simulink model "uav_with_flc_optimized_by_ga"  (R2025b)
settings: Solver=ode45  StartTime=0.0  StopTime=30  FixedStep=0.01  RelTol=1e-3
undefined symbols (not defined in the file): Ax, Ay, Az, b, d, g, Ixx, Iyy, Izz, Jr, k1_phi, k1_psi, k1_theta, k1_x, k1_y, k1_z, k2_phi, k2_psi, k2_theta, k2_x, k2_y, k2_z, Kout_phi, Kout_theta, Kout_x, Kout_y, Kout_z, L, m, omega_max, phi_ref_max, theta_ref_max, U1_max, U1_min, U2_max, U3_max, U4_max
libraries: fuzblock x6
settings Model: SimulationMode=accelerator  Creator=pc  LastModifiedBy=pc

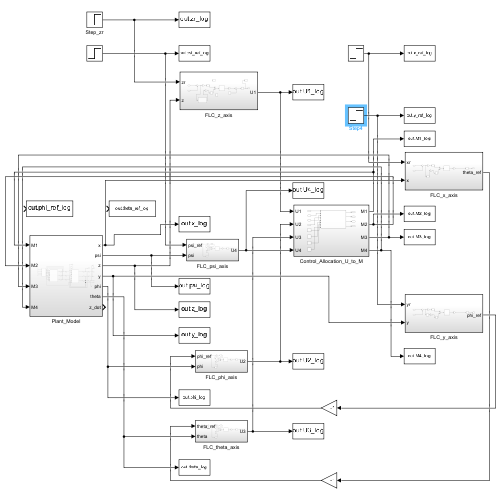
[thumbnail: Simulink's stored preview of the top-level diagram]
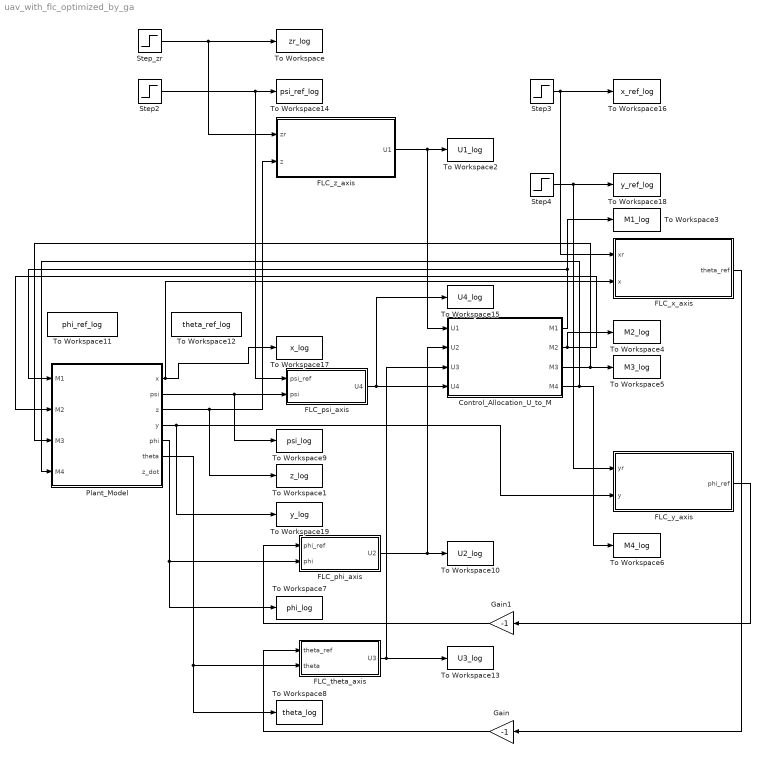
== system uav_with_flc_optimized_by_ga ==
  Control_Allocation_U_to_M : Subsystem
  FLC_phi_axis : Subsystem
  FLC_psi_axis : Subsystem
  FLC_theta_axis : Subsystem
  FLC_x_axis : Subsystem
  FLC_y_axis : Subsystem
  FLC_z_axis : Subsystem
  Gain : Gain  Gain=-1
  Gain1 : Gain  Gain=-1
  Plant_Model : Subsystem
  Step2 : Step  Time=5  After=0  SampleTime=0
  Step3 : Step  Time=10  After=0.2  SampleTime=0
  Step4 : Step  Time=10  After=0.2  SampleTime=0
  Step_zr : Step  SampleTime=0
  To Workspace : ToWorkspace  VariableName=zr_log  SaveFormat=Timeseries  SampleTime=-1
  To Workspace1 : ToWorkspace  VariableName=z_log  SaveFormat=Timeseries  SampleTime=-1
  To Workspace10 : ToWorkspace  VariableName=U2_log  SaveFormat=Timeseries  SampleTime=-1
  To Workspace11 : ToWorkspace  VariableName=phi_ref_log  SaveFormat=Timeseries  SampleTime=-1
  To Workspace12 : ToWorkspace  VariableName=theta_ref_log  SaveFormat=Timeseries  SampleTime=-1
  To Workspace13 : ToWorkspace  VariableName=U3_log  SaveFormat=Timeseries  SampleTime=-1
  To Workspace14 : ToWorkspace  VariableName=psi_ref_log  SaveFormat=Timeseries  SampleTime=-1
  To Workspace15 : ToWorkspace  VariableName=U4_log  SaveFormat=Timeseries  SampleTime=-1
  To Workspace16 : ToWorkspace  VariableName=x_ref_log  SaveFormat=Timeseries  SampleTime=-1
  To Workspace17 : ToWorkspace  VariableName=x_log  SaveFormat=Timeseries  SampleTime=-1
  To Workspace18 : ToWorkspace  VariableName=y_ref_log  SaveFormat=Timeseries  SampleTime=-1
  To Workspace19 : ToWorkspace  VariableName=y_log  SaveFormat=Timeseries  SampleTime=-1
  To Workspace2 : ToWorkspace  VariableName=U1_log  SaveFormat=Timeseries  SampleTime=-1
  To Workspace3 : ToWorkspace  VariableName=M1_log  SaveFormat=Timeseries  SampleTime=-1
  To Workspace4 : ToWorkspace  VariableName=M2_log  SaveFormat=Timeseries  SampleTime=-1
  To Workspace5 : ToWorkspace  VariableName=M3_log  SaveFormat=Timeseries  SampleTime=-1
  To Workspace6 : ToWorkspace  VariableName=M4_log  SaveFormat=Timeseries  SampleTime=-1
  To Workspace7 : ToWorkspace  VariableName=phi_log  SaveFormat=Timeseries  SampleTime=-1
  To Workspace8 : ToWorkspace  VariableName=theta_log  SaveFormat=Timeseries  SampleTime=-1
  To Workspace9 : ToWorkspace  VariableName=psi_log  SaveFormat=Timeseries  SampleTime=-1
  wires:
  Step_zr/1 -> To Workspace/1, FLC_z_axis/1(zr)
  Step2/1 -> FLC_psi_axis/1(psi_ref), To Workspace14/1
  Plant_Model/6(theta) -> To Workspace8/1, FLC_theta_axis/2(theta)
  Plant_Model/5(phi) -> FLC_phi_axis/2(phi), To Workspace7/1
  FLC_psi_axis/1(U4) -> Control_Allocation_U_to_M/4(U4), To Workspace15/1
  Plant_Model/4(y) -> FLC_y_axis/2(y), To Workspace19/1
  Step3/1 -> FLC_x_axis/1(xr), To Workspace16/1
  Plant_Model/3(z) -> To Workspace1/1, FLC_z_axis/2(z)
  Plant_Model/2(psi) -> To Workspace9/1, FLC_psi_axis/2(psi)
  Plant_Model/1(x) -> FLC_x_axis/2(x), To Workspace17/1
  FLC_z_axis/1(U1) -> To Workspace2/1, Control_Allocation_U_to_M/1(U1)
  FLC_phi_axis/1(U2) -> To Workspace10/1, Control_Allocation_U_to_M/2(U2)
  FLC_y_axis/1(phi_ref) -> Gain1/1
  FLC_theta_axis/1(U3) -> To Workspace13/1, Control_Allocation_U_to_M/3(U3)
  Gain1/1 -> FLC_phi_axis/1(phi_ref)
  Gain/1 -> FLC_theta_axis/1(theta_ref)
  Control_Allocation_U_to_M/3(M3) -> Plant_Model/3(M3), To Workspace5/1
  Step4/1 -> FLC_y_axis/1(yr), To Workspace18/1
  Control_Allocation_U_to_M/1(M1) -> Plant_Model/1(M1), To Workspace3/1
  Control_Allocation_U_to_M/2(M2) -> To Workspace4/1, Plant_Model/2(M2)
  Control_Allocation_U_to_M/4(M4) -> Plant_Model/4(M4), To Workspace6/1
  FLC_x_axis/1(theta_ref) -> Gain/1

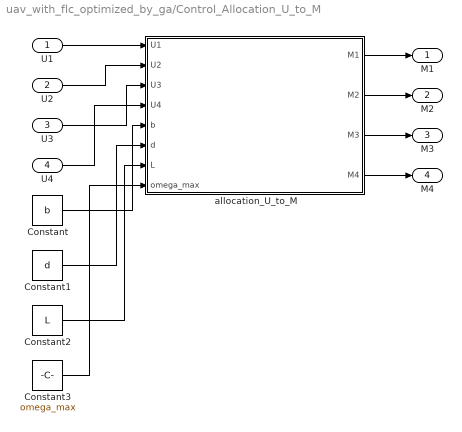
== system uav_with_flc_optimized_by_ga/Control_Allocation_U_to_M ==
  U1 : Inport
  U2 : Inport  Port=2
  U3 : Inport  Port=3
  U4 : Inport  Port=4
  Constant : Constant  Value=b
  Constant1 : Constant  Value=d
  Constant2 : Constant  Value=L
  Constant3 : Constant  Value=omega_max
  allocation_U_to_M : MATLAB Function  TreatAsAtomicUnit=on
  M1 : Outport
  M2 : Outport  Port=2
  M3 : Outport  Port=3
  M4 : Outport  Port=4
  wires:
  U1/1 -> allocation_U_to_M/1(U1)
  U2/1 -> allocation_U_to_M/2(U2)
  U3/1 -> allocation_U_to_M/3(U3)
  U4/1 -> allocation_U_to_M/4(U4)
  Constant/1 -> allocation_U_to_M/5(b)
  Constant1/1 -> allocation_U_to_M/6(d)
  Constant2/1 -> allocation_U_to_M/7(L)
  Constant3/1 -> allocation_U_to_M/8(omega_max)
  allocation_U_to_M/1(M1) -> M1/1
  allocation_U_to_M/2(M2) -> M2/1
  allocation_U_to_M/3(M3) -> M3/1
  allocation_U_to_M/4(M4) -> M4/1

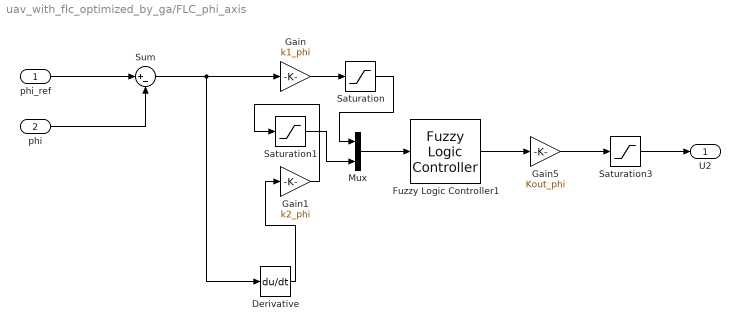
== system uav_with_flc_optimized_by_ga/FLC_phi_axis ==
  phi_ref : Inport
  phi : Inport  Port=2
  Derivative : Derivative
  Fuzzy Logic Controller1 : fuzblock/Fuzzy Logic  Controller  FIS=fis_axis  OutputSampleNumber=101  DataType=double  UseLookupTable=off  NumBreakpoints=10  FuzzifiedInputs=off  RuleFiringStrengths=off  RuleOutputs=off  AggregatedOutputs=off  SimulateUsing=Interpreted execution  OutOfRangeInputValueMessage=warning  NoRuleFiredMessage=warning  EmptyOutputFuzzySetMessage=warning
  Gain : Gain  Gain=k1_phi
  Gain1 : Gain  Gain=k2_phi
  Gain5 : Gain  Gain=Kout_phi
  Mux : Mux  Inputs=2
  Saturation : Saturate  UpperLimit=1  LowerLimit=-1  ZeroCross=off
  Saturation1 : Saturate  UpperLimit=1  LowerLimit=-1  ZeroCross=off
  Saturation3 : Saturate  UpperLimit=U2_max  LowerLimit=-U2_max
  Sum : Sum  Inputs=|+-
  U2 : Outport
  wires:
  phi_ref/1 -> Sum/1
  phi/1 -> Sum/2
  Derivative/1 -> Gain1/1
  Sum/1 -> Derivative/1, Gain/1
  Mux/1 -> Fuzzy Logic Controller1/1
  Fuzzy Logic Controller1/1 -> Gain5/1
  Gain5/1 -> Saturation3/1
  Saturation3/1 -> U2/1
  Gain/1 -> Saturation/1
  Saturation/1 -> Mux/1
  Gain1/1 -> Saturation1/1
  Saturation1/1 -> Mux/2

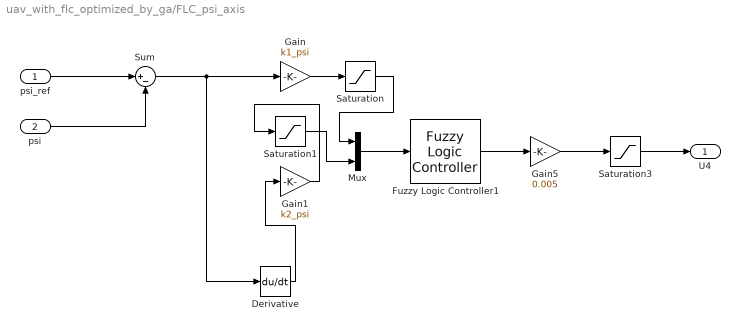
== system uav_with_flc_optimized_by_ga/FLC_psi_axis ==
  psi_ref : Inport
  psi : Inport  Port=2
  Derivative : Derivative
  Fuzzy Logic Controller1 : fuzblock/Fuzzy Logic  Controller  FIS=fis_axis  OutputSampleNumber=101  DataType=double  UseLookupTable=off  NumBreakpoints=10  FuzzifiedInputs=off  RuleFiringStrengths=off  RuleOutputs=off  AggregatedOutputs=off  SimulateUsing=Interpreted execution  OutOfRangeInputValueMessage=warning  NoRuleFiredMessage=warning  EmptyOutputFuzzySetMessage=warning
  Gain : Gain  Gain=k1_psi
  Gain1 : Gain  Gain=k2_psi
  Gain5 : Gain  Gain=0.005
  Mux : Mux  Inputs=2
  Saturation : Saturate  UpperLimit=1  LowerLimit=-1  ZeroCross=off
  Saturation1 : Saturate  UpperLimit=1  LowerLimit=-1  ZeroCross=off
  Saturation3 : Saturate  UpperLimit=U4_max  LowerLimit=-U4_max
  Sum : Sum  Inputs=|+-
  U4 : Outport
  wires:
  psi_ref/1 -> Sum/1
  psi/1 -> Sum/2
  Derivative/1 -> Gain1/1
  Sum/1 -> Derivative/1, Gain/1
  Mux/1 -> Fuzzy Logic Controller1/1
  Fuzzy Logic Controller1/1 -> Gain5/1
  Gain5/1 -> Saturation3/1
  Saturation3/1 -> U4/1
  Gain/1 -> Saturation/1
  Saturation/1 -> Mux/1
  Gain1/1 -> Saturation1/1
  Saturation1/1 -> Mux/2

== system uav_with_flc_optimized_by_ga/FLC_theta_axis ==
  theta_ref : Inport
  theta : Inport  Port=2
  Derivative : Derivative
  Fuzzy Logic Controller1 : fuzblock/Fuzzy Logic  Controller  FIS=fis_axis  OutputSampleNumber=101  DataType=double  UseLookupTable=off  NumBreakpoints=10  FuzzifiedInputs=off  RuleFiringStrengths=off  RuleOutputs=off  AggregatedOutputs=off  SimulateUsing=Interpreted execution  OutOfRangeInputValueMessage=warning  NoRuleFiredMessage=warning  EmptyOutputFuzzySetMessage=warning
  Gain : Gain  Gain=k1_theta
  Gain1 : Gain  Gain=k2_theta
  Gain5 : Gain  Gain=Kout_theta
  Mux : Mux  Inputs=2
  Saturation : Saturate  UpperLimit=1  LowerLimit=-1  ZeroCross=off
  Saturation1 : Saturate  UpperLimit=1  LowerLimit=-1  ZeroCross=off
  Saturation3 : Saturate  UpperLimit=U3_max  LowerLimit=-U3_max
  Sum : Sum  Inputs=|+-
  U3 : Outport
  wires:
  theta_ref/1 -> Sum/1
  theta/1 -> Sum/2
  Derivative/1 -> Gain1/1
  Sum/1 -> Derivative/1, Gain/1
  Mux/1 -> Fuzzy Logic Controller1/1
  Fuzzy Logic Controller1/1 -> Gain5/1
  Gain5/1 -> Saturation3/1
  Saturation3/1 -> U3/1
  Gain/1 -> Saturation/1
  Saturation/1 -> Mux/1
  Gain1/1 -> Saturation1/1
  Saturation1/1 -> Mux/2

== system uav_with_flc_optimized_by_ga/FLC_x_axis ==
  xr : Inport
  x : Inport  Port=2
  Derivative : Derivative
  Fuzzy Logic Controller : fuzblock/Fuzzy Logic  Controller  FIS=fis_axis  OutputSampleNumber=101  DataType=double  UseLookupTable=off  NumBreakpoints=10  FuzzifiedInputs=off  RuleFiringStrengths=off  RuleOutputs=off  AggregatedOutputs=off  SimulateUsing=Interpreted execution  OutOfRangeInputValueMessage=warning  NoRuleFiredMessage=warning  EmptyOutputFuzzySetMessage=warning
  Gain : Gain  Gain=k1_x
  Gain1 : Gain  Gain=k2_x
  Gain2 : Gain  Gain=Kout_x
  Mux : Mux  Inputs=2
  Saturation : Saturate  UpperLimit=theta_ref_max  LowerLimit=-theta_ref_max
  Saturation1 : Saturate  UpperLimit=0.95  LowerLimit=-0.95  ZeroCross=off
  Saturation2 : Saturate  UpperLimit=0.95  LowerLimit=-0.95  ZeroCross=off
  Sum : Sum  Inputs=|+-
  theta_ref : Outport
  wires:
  xr/1 -> Sum/1
  x/1 -> Sum/2
  Sum/1 -> Derivative/1, Gain/1
  Gain/1 -> Saturation1/1
  Gain1/1 -> Saturation2/1
  Mux/1 -> Fuzzy Logic Controller/1
  Fuzzy Logic Controller/1 -> Gain2/1
  Saturation/1 -> theta_ref/1
  Gain2/1 -> Saturation/1
  Saturation1/1 -> Mux/1
  Derivative/1 -> Gain1/1
  Saturation2/1 -> Mux/2

== system uav_with_flc_optimized_by_ga/FLC_y_axis ==
  yr : Inport
  y : Inport  Port=2
  Derivative : Derivative
  Fuzzy Logic Controller : fuzblock/Fuzzy Logic  Controller  FIS=fis_axis  OutputSampleNumber=101  DataType=double  UseLookupTable=off  NumBreakpoints=10  FuzzifiedInputs=off  RuleFiringStrengths=off  RuleOutputs=off  AggregatedOutputs=off  SimulateUsing=Interpreted execution  OutOfRangeInputValueMessage=warning  NoRuleFiredMessage=warning  EmptyOutputFuzzySetMessage=warning
  Gain : Gain  Gain=k1_y
  Gain1 : Gain  Gain=k2_y
  Gain2 : Gain  Gain=Kout_y
  Mux : Mux  Inputs=2
  Saturation : Saturate  UpperLimit=phi_ref_max  LowerLimit=-phi_ref_max
  Saturation1 : Saturate  UpperLimit=0.95  LowerLimit=-0.95  ZeroCross=off
  Saturation2 : Saturate  UpperLimit=0.95  LowerLimit=-0.95  ZeroCross=off
  Sum : Sum  Inputs=|+-
  phi_ref : Outport
  wires:
  yr/1 -> Sum/1
  y/1 -> Sum/2
  Sum/1 -> Derivative/1, Gain/1
  Gain/1 -> Saturation1/1
  Gain1/1 -> Saturation2/1
  Mux/1 -> Fuzzy Logic Controller/1
  Fuzzy Logic Controller/1 -> Gain2/1
  Saturation/1 -> phi_ref/1
  Gain2/1 -> Saturation/1
  Saturation1/1 -> Mux/1
  Derivative/1 -> Gain1/1
  Saturation2/1 -> Mux/2

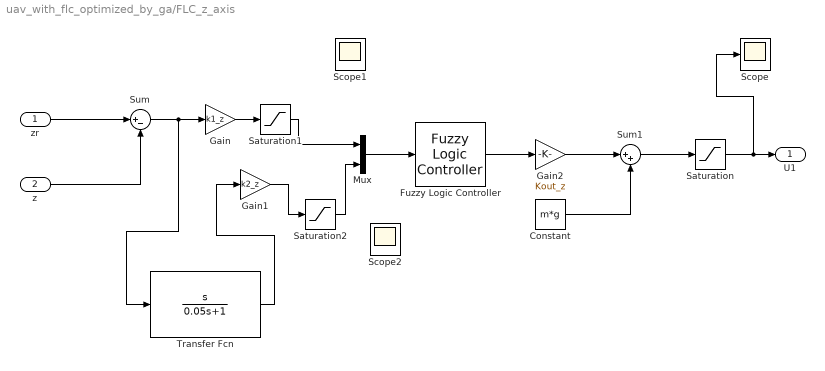
== system uav_with_flc_optimized_by_ga/FLC_z_axis ==
  zr : Inport
  z : Inport  Port=2
  Constant : Constant  Value=m*g
  Fuzzy Logic Controller : fuzblock/Fuzzy Logic  Controller  FIS=fis_axis  OutputSampleNumber=101  DataType=double  UseLookupTable=off  NumBreakpoints=10  FuzzifiedInputs=off  RuleFiringStrengths=off  RuleOutputs=off  AggregatedOutputs=off  SimulateUsing=Interpreted execution  OutOfRangeInputValueMessage=warning  NoRuleFiredMessage=warning  EmptyOutputFuzzySetMessage=warning
  Gain : Gain  Gain=k1_z
  Gain1 : Gain  Gain=k2_z
  Gain2 : Gain  Gain=Kout_z
  Mux : Mux  Inputs=2
  Saturation : Saturate  UpperLimit=U1_max  LowerLimit=U1_min
  Saturation1 : Saturate  UpperLimit=0.99  LowerLimit=-0.99  ZeroCross=off
  Saturation2 : Saturate  UpperLimit=0.99  LowerLimit=-0.99  ZeroCross=off
  Scope : Scope
      settings: ActiveDisplayYMinimum=-5.3947101328264253  ActiveDisplayYMaximum=19.82403131441027  DataLoggingVariableName=ScopeData3
  Scope1 : Scope
      settings: ActiveDisplayYMinimum=-1.8162957380086806  ActiveDisplayYMaximum=2.2569101049179121  DataLoggingVariableName=ScopeData13
  Scope2 : Scope
      settings: ActiveDisplayYMinimum=-1.3687471275725305  ActiveDisplayYMaximum=1.5167298507169844  DataLoggingVariableName=ScopeData14
  Sum : Sum  Inputs=|+-
  Sum1 : Sum  Inputs=|++
  Transfer Fcn : TransferFcn  Numerator=[1 0]  Denominator=[0.05 1]
  U1 : Outport
  wires:
  zr/1 -> Sum/1
  z/1 -> Sum/2
  Sum/1 -> Transfer Fcn/1, Gain/1
  Gain/1 -> Saturation1/1
  Gain1/1 -> Saturation2/1
  Mux/1 -> Fuzzy Logic Controller/1
  Fuzzy Logic Controller/1 -> Gain2/1
  Gain2/1 -> Sum1/1
  Constant/1 -> Sum1/2
  Saturation/1 -> Scope/1, U1/1
  Sum1/1 -> Saturation/1
  Saturation1/1 -> Mux/1
  Transfer Fcn/1 -> Gain1/1
  Saturation2/1 -> Mux/2

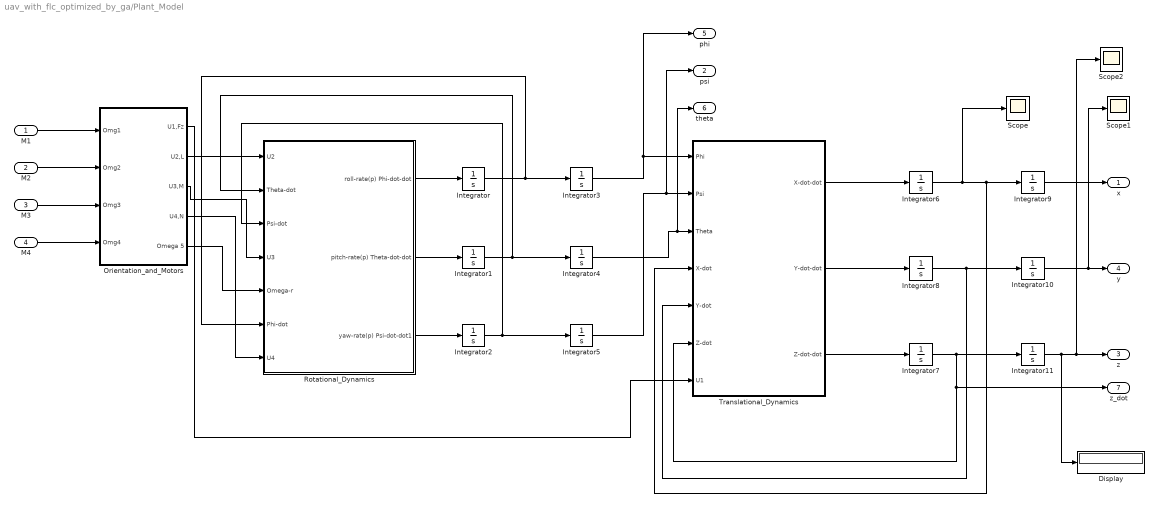
== system uav_with_flc_optimized_by_ga/Plant_Model ==
  M1 : Inport
  M2 : Inport  Port=2
  M3 : Inport  Port=3
  M4 : Inport  Port=4
  Display : Display
  Integrator{,1..2,6..10} (8 alike) : Integrator
  Integrator11 : Integrator  LimitOutput=on  LowerSaturationLimit=0
  Integrator3 : Integrator  WrapState=on
  Integrator4 : Integrator  WrapState=on
  Integrator5 : Integrator  WrapState=on
  Orientation_and_Motors : Subsystem
  Rotational_Dynamics : Subsystem
  Scope : Scope
      settings: ActiveDisplayYMinimum=-1.7548410090540747  ActiveDisplayYMaximum=1.5029482445008098
  Scope1 : Scope
      settings: ActiveDisplayYMinimum=-2.9564597824624426  ActiveDisplayYMaximum=1.6275768531396264
  Scope2 : Scope
      settings: ActiveDisplayYMinimum=-1622.417766731558  ActiveDisplayYMaximum=231.6352006550556  DataLoggingVariableName=ScopeData2
  Translational_Dynamics : Subsystem
  x : Outport
  psi : Outport  Port=2
  z : Outport  Port=3
  y : Outport  Port=4
  phi : Outport  Port=5
  theta : Outport  Port=6
  z_dot : Outport  Port=7
  wires:
  M1/1 -> Orientation_and_Motors/1(Omg1)
  M2/1 -> Orientation_and_Motors/2(Omg2)
  M3/1 -> Orientation_and_Motors/3(Omg3)
  M4/1 -> Orientation_and_Motors/4(Omg4)
  Orientation_and_Motors/2(U2,L) -> Rotational_Dynamics/1(U2)
  Orientation_and_Motors/3(U3,M) -> Rotational_Dynamics/4(U3)
  Orientation_and_Motors/4(U4,N) -> Rotational_Dynamics/7(U4)
  Orientation_and_Motors/5(Omega 5) -> Rotational_Dynamics/5(Omega-r)
  Rotational_Dynamics/1(roll-rate(p) Phi-dot-dot) -> Integrator/1
  Rotational_Dynamics/2(pitch-rate(p) Theta-dot-dot) -> Integrator1/1
  Rotational_Dynamics/3(yaw-rate(p) Psi-dot-dot1) -> Integrator2/1
  Integrator/1 -> Integrator3/1, Rotational_Dynamics/6(Phi-dot)
  Integrator1/1 -> Integrator4/1, Rotational_Dynamics/2(Theta-dot)
  Integrator2/1 -> Integrator5/1, Rotational_Dynamics/3(Psi-dot)
  Integrator3/1 -> phi/1, Translational_Dynamics/1(Phi)
  Integrator5/1 -> psi/1, Translational_Dynamics/2(Psi)
  Integrator4/1 -> theta/1, Translational_Dynamics/3(Theta)
  Translational_Dynamics/1(X-dot-dot) -> Integrator6/1
  Translational_Dynamics/3(Z-dot-dot) -> Integrator7/1
  Translational_Dynamics/2(Y-dot-dot) -> Integrator8/1
  Integrator6/1 -> Translational_Dynamics/4(X-dot), Integrator9/1, Scope/1
  Integrator7/1 -> z_dot/1, Translational_Dynamics/6(Z-dot), Integrator11/1
  Integrator8/1 -> Translational_Dynamics/5(Y-dot), Integrator10/1
  Orientation_and_Motors/1(U1,Fz) -> Translational_Dynamics/7(U1)
  Integrator10/1 -> Scope1/1, y/1
  Integrator9/1 -> x/1
  Integrator11/1 -> Display/1, z/1, Scope2/1

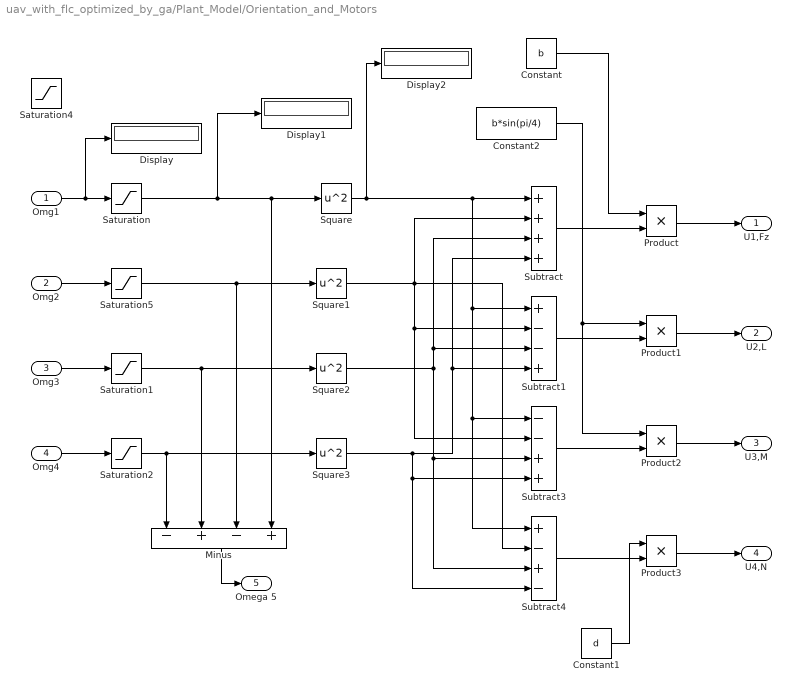
== system uav_with_flc_optimized_by_ga/Plant_Model/Orientation_and_Motors ==
  Omg1 : Inport
  Omg2 : Inport  Port=2
  Omg3 : Inport  Port=3
  Omg4 : Inport  Port=4
  Constant : Constant  Value=b
  Constant1 : Constant  Value=d
  Constant2 : Constant  Value=b*sin(pi/4)
  Display : Display
  Display1 : Display
  Display2 : Display
  Minus : Sum  Inputs=-+-+
  Product{,1..3} (4 alike) : Product
  Saturation{,1..2,5} (4 alike) : Saturate  UpperLimit=omega_max  LowerLimit=0
  Saturation4 : Saturate
  Square{,1..3} (4 alike) : Math  Operator=square
  Subtract : Sum  Inputs=++++
  Subtract1 : Sum  Inputs=+--+
  Subtract3 : Sum  Inputs=--++
  Subtract4 : Sum  Inputs=+-+-
  U1,Fz : Outport
  U2,L : Outport  Port=2
  U3,M : Outport  Port=3
  U4,N : Outport  Port=4
  Omega 5 : Outport  Port=5
  wires:
  Omg1/1 -> Display/1, Saturation/1
  Omg2/1 -> Saturation5/1
  Omg3/1 -> Saturation1/1
  Omg4/1 -> Saturation2/1
  Saturation/1 -> Display1/1, Minus/4, Square/1
  Saturation1/1 -> Minus/2, Square2/1
  Saturation2/1 -> Minus/1, Square3/1
  Saturation5/1 -> Minus/3, Square1/1
  Minus/1 -> Omega 5/1
  Square/1 -> Subtract4/1, Subtract3/1, Subtract1/1, Subtract/1, Display2/1
  Square1/1 -> Subtract4/2, Subtract3/2, Subtract1/2, Subtract/2
  Square2/1 -> Subtract4/3, Subtract3/3, Subtract1/3, Subtract/3
  Square3/1 -> Subtract4/4, Subtract3/4, Subtract1/4, Subtract/4
  Subtract/1 -> Product/2
  Constant/1 -> Product/1
  Product/1 -> U1,Fz/1
  Subtract1/1 -> Product1/2
  Constant2/1 -> Product2/1, Product1/1
  Subtract3/1 -> Product2/2
  Product1/1 -> U2,L/1
  Product2/1 -> U3,M/1
  Subtract4/1 -> Product3/2
  Constant1/1 -> Product3/1
  Product3/1 -> U4,N/1

== system uav_with_flc_optimized_by_ga/Plant_Model/Rotational_Dynamics ==
  note: Roll Angle Acceleration Subsystem
  note: Pitch Angle Acceleration Subsystem
  note: Yaw Angle Acceleration Subsystem
  U2 : Inport
  Theta-dot : Inport  Port=2
  Psi-dot : Inport  Port=3
  U3 : Inport  Port=4
  Omega-r : Inport  Port=5
  Phi-dot : Inport  Port=6
  U4 : Inport  Port=7
  pitch-angl-acc : Subsystem
  roll-angl-acc : Subsystem
  yaw-angl-acc : Subsystem
  roll-rate(p) Phi-dot-dot : Outport
  pitch-rate(p) Theta-dot-dot : Outport  Port=2
  yaw-rate(p) Psi-dot-dot1 : Outport  Port=3
  wires:
  U2/1 -> roll-angl-acc/1(U2)
  Omega-r/1 -> pitch-angl-acc/2(Omega-r), roll-angl-acc/2(Omega-r)
  U3/1 -> pitch-angl-acc/1(U3)
  Psi-dot/1 -> pitch-angl-acc/4(Psi-dot), roll-angl-acc/4(Psi-dot)
  Theta-dot/1 -> roll-angl-acc/3(Theta-dot), yaw-angl-acc/2(Theta-dot)
  Phi-dot/1 -> yaw-angl-acc/3(Phi-dot), pitch-angl-acc/3(Phi-dot)
  U4/1 -> yaw-angl-acc/1(U4)
  roll-angl-acc/1(Phi-dot-dot) -> roll-rate(p) Phi-dot-dot/1
  yaw-angl-acc/1(Psi-dot-dot) -> yaw-rate(p) Psi-dot-dot1/1
  pitch-angl-acc/1(Theta-dot-dot) -> pitch-rate(p) Theta-dot-dot/1

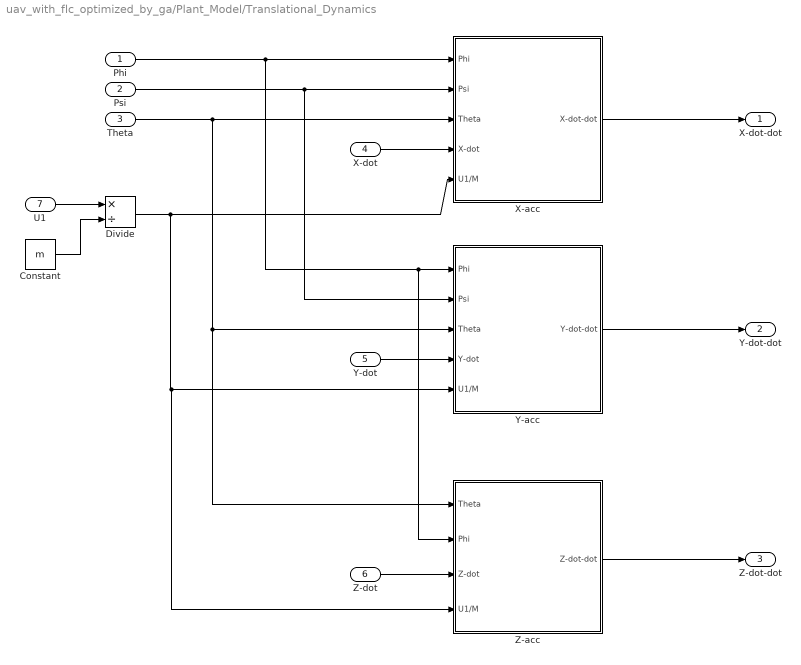
== system uav_with_flc_optimized_by_ga/Plant_Model/Translational_Dynamics ==
  Phi : Inport
  Psi : Inport  Port=2
  Theta : Inport  Port=3
  X-dot : Inport  Port=4
  Y-dot : Inport  Port=5
  Z-dot : Inport  Port=6
  U1 : Inport  Port=7
  Constant : Constant  Value=m
  Divide : Product  Inputs=*/
  X-acc : Subsystem
  Y-acc : Subsystem
  Z-acc : Subsystem
  X-dot-dot : Outport
  Y-dot-dot : Outport  Port=2
  Z-dot-dot : Outport  Port=3
  wires:
  Phi/1 -> Z-acc/2(Phi), Y-acc/1(Phi), X-acc/1(Phi)
  Psi/1 -> Y-acc/2(Psi), X-acc/2(Psi)
  Theta/1 -> Z-acc/1(Theta), Y-acc/3(Theta), X-acc/3(Theta)
  X-dot/1 -> X-acc/4(X-dot)
  U1/1 -> Divide/1
  Constant/1 -> Divide/2
  Divide/1 -> Z-acc/4(U1/M), Y-acc/5(U1/M), X-acc/5(U1/M)
  Y-dot/1 -> Y-acc/4(Y-dot)
  Y-acc/1(Y-dot-dot) -> Y-dot-dot/1
  X-acc/1(X-dot-dot) -> X-dot-dot/1
  Z-dot/1 -> Z-acc/3(Z-dot)
  Z-acc/1(Z-dot-dot) -> Z-dot-dot/1

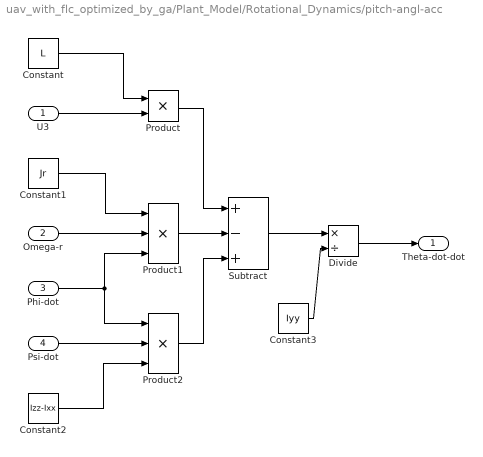
== system uav_with_flc_optimized_by_ga/Plant_Model/Rotational_Dynamics/pitch-angl-acc ==
  U3 : Inport
  Omega-r : Inport  Port=2
  Phi-dot : Inport  Port=3
  Psi-dot : Inport  Port=4
  Constant : Constant  Value=L
  Constant1 : Constant  Value=Jr
  Constant2 : Constant  Value=Izz-Ixx
  Constant3 : Constant  Value=Iyy
  Divide : Product  Inputs=*/
  Product : Product
  Product1 : Product  Inputs=3
  Product2 : Product  Inputs=3
  Subtract : Sum  Inputs=+-+
  Theta-dot-dot : Outport
  wires:
  U3/1 -> Product/2
  Constant/1 -> Product/1
  Omega-r/1 -> Product1/2
  Constant1/1 -> Product1/1
  Phi-dot/1 -> Product2/1, Product1/3
  Psi-dot/1 -> Product2/2
  Constant2/1 -> Product2/3
  Product1/1 -> Subtract/2
  Product/1 -> Subtract/1
  Product2/1 -> Subtract/3
  Subtract/1 -> Divide/1
  Constant3/1 -> Divide/2
  Divide/1 -> Theta-dot-dot/1

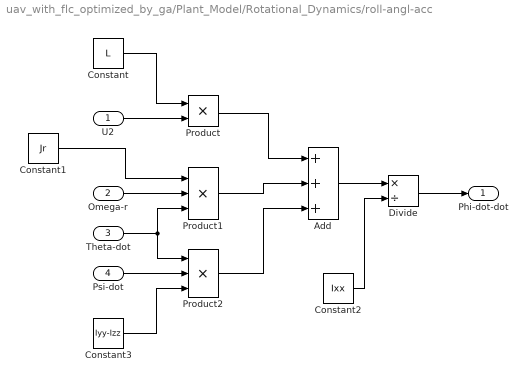
== system uav_with_flc_optimized_by_ga/Plant_Model/Rotational_Dynamics/roll-angl-acc ==
  U2 : Inport
  Omega-r : Inport  Port=2
  Theta-dot : Inport  Port=3
  Psi-dot : Inport  Port=4
  Add : Sum  Inputs=+++
  Constant : Constant  Value=L
  Constant1 : Constant  Value=Jr
  Constant2 : Constant  Value=Ixx
  Constant3 : Constant  Value=Iyy-Izz
  Divide : Product  Inputs=*/
  Product : Product
  Product1 : Product  Inputs=3
  Product2 : Product  Inputs=3
  Phi-dot-dot : Outport
  wires:
  U2/1 -> Product/2
  Constant/1 -> Product/1
  Product/1 -> Add/1
  Product1/1 -> Add/2
  Omega-r/1 -> Product1/2
  Product2/1 -> Add/3
  Add/1 -> Divide/1
  Divide/1 -> Phi-dot-dot/1
  Constant2/1 -> Divide/2
  Psi-dot/1 -> Product2/2
  Theta-dot/1 -> Product1/3, Product2/1
  Constant3/1 -> Product2/3
  Constant1/1 -> Product1/1

== system uav_with_flc_optimized_by_ga/Plant_Model/Rotational_Dynamics/yaw-angl-acc ==
  U4 : Inport
  Theta-dot : Inport  Port=2
  Phi-dot : Inport  Port=3
  Constant : Constant  Value=Ixx-Iyy
  Constant1 : Constant  Value=Izz
  Divide : Product  Inputs=*/
  Product : Product  Inputs=3
  Subtract : Sum
  Psi-dot-dot : Outport
  wires:
  Theta-dot/1 -> Product/1
  Phi-dot/1 -> Product/2
  Constant/1 -> Product/3
  U4/1 -> Subtract/1
  Product/1 -> Subtract/2
  Subtract/1 -> Divide/1
  Constant1/1 -> Divide/2
  Divide/1 -> Psi-dot-dot/1

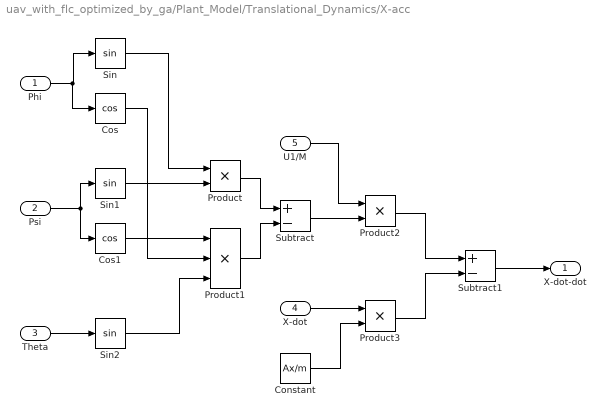
== system uav_with_flc_optimized_by_ga/Plant_Model/Translational_Dynamics/X-acc ==
  Phi : Inport
  Psi : Inport  Port=2
  Theta : Inport  Port=3
  X-dot : Inport  Port=4
  U1/M : Inport  Port=5
  Constant : Constant  Value=Ax/m
  Cos : Trigonometry  Operator=cos
  Cos1 : Trigonometry  Operator=cos
  Product : Product
  Product1 : Product  Inputs=3
  Product2 : Product
  Product3 : Product
  Sin : Trigonometry
  Sin1 : Trigonometry
  Sin2 : Trigonometry
  Subtract : Sum  Inputs=+-
  Subtract1 : Sum  Inputs=+-
  X-dot-dot : Outport
  wires:
  Phi/1 -> Cos/1, Sin/1
  Psi/1 -> Cos1/1, Sin1/1
  Theta/1 -> Sin2/1
  Sin1/1 -> Product/2
  Sin/1 -> Product/1
  Cos/1 -> Product1/2
  Cos1/1 -> Product1/1
  Sin2/1 -> Product1/3
  Product/1 -> Subtract/1
  Product1/1 -> Subtract/2
  Subtract/1 -> Product2/2
  U1/M/1 -> Product2/1
  X-dot/1 -> Product3/1
  Product2/1 -> Subtract1/1
  Product3/1 -> Subtract1/2
  Subtract1/1 -> X-dot-dot/1
  Constant/1 -> Product3/2

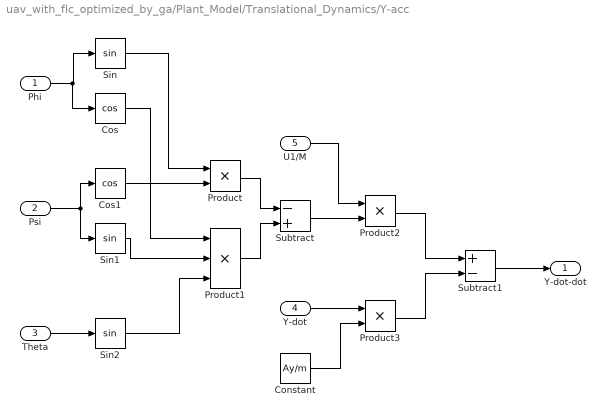
== system uav_with_flc_optimized_by_ga/Plant_Model/Translational_Dynamics/Y-acc ==
  Phi : Inport
  Psi : Inport  Port=2
  Theta : Inport  Port=3
  Y-dot : Inport  Port=4
  U1/M : Inport  Port=5
  Constant : Constant  Value=Ay/m
  Cos : Trigonometry  Operator=cos
  Cos1 : Trigonometry  Operator=cos
  Product : Product
  Product1 : Product  Inputs=3
  Product2 : Product
  Product3 : Product
  Sin : Trigonometry
  Sin1 : Trigonometry
  Sin2 : Trigonometry
  Subtract : Sum  Inputs=-+
  Subtract1 : Sum  Inputs=+-
  Y-dot-dot : Outport
  wires:
  Product3/1 -> Subtract1/2
  Constant/1 -> Product3/2
  Subtract1/1 -> Y-dot-dot/1
  Product2/1 -> Subtract1/1
  Product1/1 -> Subtract/2
  Sin/1 -> Product/1
  Phi/1 -> Cos/1, Sin/1
  Subtract/1 -> Product2/2
  Psi/1 -> Sin1/1, Cos1/1
  Product/1 -> Subtract/1
  Theta/1 -> Sin2/1
  U1/M/1 -> Product2/1
  Y-dot/1 -> Product3/1
  Sin2/1 -> Product1/3
  Cos1/1 -> Product/2
  Sin1/1 -> Product1/2
  Cos/1 -> Product1/1

== system uav_with_flc_optimized_by_ga/Plant_Model/Translational_Dynamics/Z-acc ==
  Theta : Inport
  Phi : Inport  Port=2
  Z-dot : Inport  Port=3
  U1/M : Inport  Port=4
  Constant : Constant  Value=Az/m
  Constant1 : Constant  Value=g
  Cos : Trigonometry  Operator=cos
  Cos1 : Trigonometry  Operator=cos
  Product : Product  Inputs=3
  Product1 : Product
  Subtract : Sum  Inputs=+-
  Subtract1 : Sum  Inputs=-+
  Z-dot-dot : Outport
  wires:
  Theta/1 -> Cos/1
  Phi/1 -> Cos1/1
  Cos1/1 -> Product/2
  Cos/1 -> Product/1
  U1/M/1 -> Product/3
  Z-dot/1 -> Product1/1
  Constant/1 -> Product1/2
  Product1/1 -> Subtract/2
  Subtract/1 -> Z-dot-dot/1
  Constant1/1 -> Subtract1/1
  Product/1 -> Subtract1/2
  Subtract1/1 -> Subtract/1

== matlab function uav_with_flc_optimized_by_ga/Control_Allocation_U_to_M/allocation_U_to_M ==
  data: U1 input; M1 output; U2 input; U3 input; U4 input; b input; d input; L input; omega_max input; M2 output; M3 output; M4 output
function [M1,M2,M3,M4] = allocation_U_to_M(U1,U2,U3,U4,b,d,L,omega_max)

arm = L/sqrt(2);

A = [ ...
    b,       b,       b,       b;
    b*arm,  -b*arm,  -b*arm,   b*arm;
   -b*arm,  -b*arm,   b*arm,   b*arm;
    d,      -d,       d,      -d];

U = [U1; U2; U3; U4];

w2 = A \ U;

% ochrana pred zápornými hodnotami
w2(1) = max(w2(1),0);
w2(2) = max(w2(2),0);
w2(3) = max(w2(3),0);
w2(4) = max(w2(4),0);

% motorové limity
w2(1) = min(w2(1),omega_max^2);
w2(2) = min(w2(2),omega_max^2);
w2(3) = min(w2(3),omega_max^2);
w2(4) = min(w2(4),omega_max^2);

M1 = sqrt(w2(1));
M2 = sqrt(w2(2));
M3 = sqrt(w2(3));
M4 = sqrt(w2(4));

end
